simulink model "Detumbling_using_engine_sim"  (R2022b)
settings: Solver=VariableStepAuto  StartTime=0.0  StopTime=Params.tf  FixedStep=1e-2  RelTol=1e-8  AbsTol=1e-8
values from neighbouring files (symbols this model uses):
  Pitch_thrust_operator = abs(-1/( (1/(norm(Params.arm_vec1)))*(sin(gamma1)*sin(theta)*Params.arm_vec1(3)-cos(gamma1)*Params.arm_vec1(1))+         (1/(norm(Params.arm_vec2)))*(-sin(gamma2)*sin(theta)*Params.arm_vec2(3)-cos(gamma2)*Params.arm_vec2(1))+         (1/(norm(Params.arm_vec3)))*(sin(gamma3)*cos(theta)*Params.arm_vec3(3)+cos(gamma3)*Params.arm_vec3(2))+         (1/(norm(Params.arm_vec4)))*(sin(gamma4)*sin(theta)*Pa ...(+61 chars)    [Detumbling_using_engine_SimCode.m]
  Roll_thrust_operator = abs(-1/( (1/(norm(Params.arm_vec1)))*(-sin(gamma1)*cos(theta)*Params.arm_vec1(3)+cos(gamma1)*Params.arm_vec1(2))+         (1/(norm(Params.arm_vec2)))*(-sin(gamma2)*cos(theta)*Params.arm_vec2(3)+cos(gamma2)*Params.arm_vec2(2))+         (1/(norm(Params.arm_vec3)))*(sin(gamma3)*sin(theta)*Params.arm_vec3(3)-cos(gamma3)*Params.arm_vec3(1))+         (1/(norm(Params.arm_vec4)))*(sin(gamma4)*cos(theta)*P ...(+51 chars)    [Detumbling_using_engine_SimCode.m]
  tau_Thrusters = 30e-03    (= 0.03)    [Detumbling_using_engine_SimCode.m]
  w_c = [0,0,0]'    [Detumbling_using_engine_SimCode.m]
  Yaw_thrust_operator = abs(-1/( (1/(norm(Params.arm_vec1)))*(-sin(gamma1)*sin(theta)*Params.arm_vec1(2)+cos(theta)*sin(gamma1)*Params.arm_vec1(1))+         (1/(norm(Params.arm_vec2)))*(-sin(gamma2)*sin(theta)*Params.arm_vec2(2)-cos(theta)*sin(gamma2)*Params.arm_vec2(1))+         (1/(norm(Params.arm_vec3)))*(-sin(gamma3)*sin(theta)*Params.arm_vec3(2)-sin(gamma3)*cos(theta)*Params.arm_vec3(1))+         (1/(norm(Params.arm ...(+86 chars)    [Detumbling_using_engine_SimCode.m]
undefined symbols (not defined in the file or in its folder): gain, Params, Pitch, rad, Roll, s, T1, time_T1, Yaw
libraries: matrix_library x24, aerolibconvert2 x1, simulink_extras x1, sharedutil x1
(part 1 of 2)
settings Model: Creator=orena  LastModifiedBy=שקד
settings SolverCC: AlgebraicLoopSolver=TrustRegion
settings DebuggingCC: UnconnectedInputMsg=warning  UnconnectedOutputMsg=warning  UnconnectedLineMsg=warning  SFMachineParentedDataDiag=warning
settings ModelReferenceCC: EnableRefExpFcnMdlSchedulingChecks=on
settings RTWCC: DLArmComputeVersion=19.05

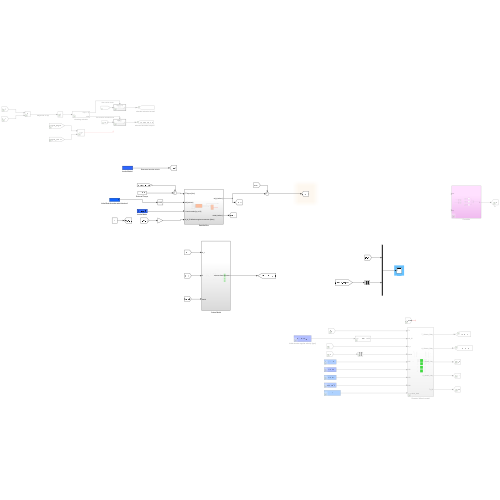
[thumbnail: Simulink's stored preview of the top-level diagram]
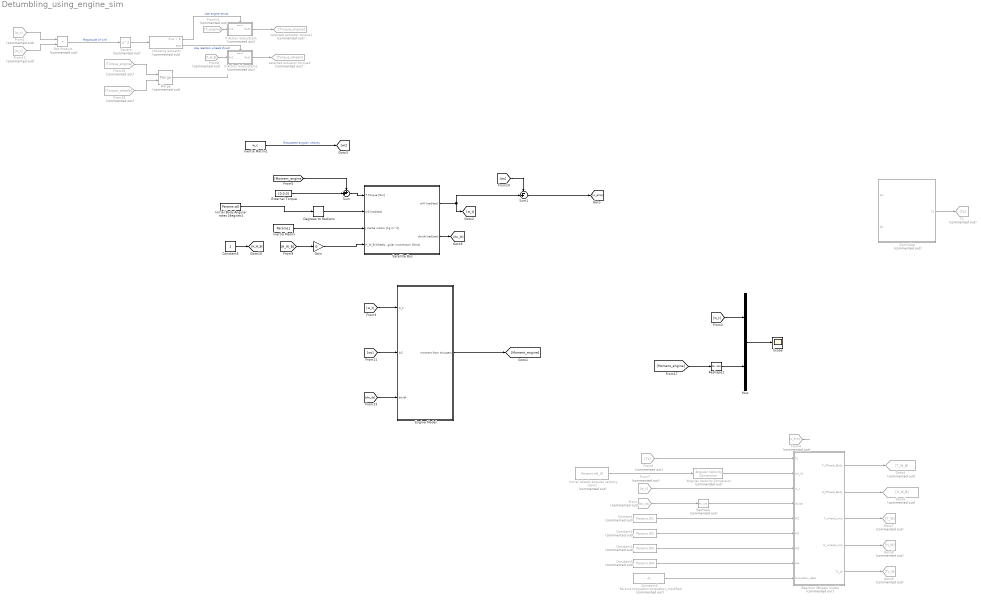
== system Detumbling_using_engine_sim ==
  Angular Velocity Conversion : aerolibconvert2/Angular Velocity Conversion  Commented=on  IU=rpm  OU=rad/s
  Constant : Constant  Commented=on  Value=Params.W1
  Constant1 : Constant  Commented=on  Value=Params.W2
  Constant2 : Constant  Commented=on  Value=Params.W3
  Constant3 : Constant  Commented=on  Value=Params.W4
  Constant4 : Constant  Commented=on  Value=Params.torquebox.torquebox_modified
  Constant5 : Constant
  Controller : Subsystem  Commented=on
  Degrees to Radians : simulink_extras/Transformations/Degrees to Radians
  Dot Product : DotProduct  Commented=on  OutDataTypeStr=Inherit: Inherit via internal rule
  Engine Model : Subsystem
  External Torque : Constant  Value=[0,0,0]
  From : From  Commented=on  GotoTag=dw_dt
  From1 : From  Commented=on  GotoTag=w_t
  From12 : From  Commented=on  GotoTag=w_t
  From14 : From  Commented=on  GotoTag=T_engine
  From15 : From  Commented=on  GotoTag=Torque_engine
  From16 : From  Commented=on  GotoTag=Torque_wheels
  From4 : From  Commented=on  GotoTag=w_error
  From6 : From  Commented=on  GotoTag=Tc
  From7 : From  Commented=on  GotoTag=w_t
  From8 : From  Commented=on  GotoTag=T_W_B
  Gain : Gain  Gain=0
  Goto4 : Goto  Commented=on  GotoTag=T_W_B
  Goto6 : Goto  Commented=on  GotoTag=H_W_B
  Goto7 : Goto  Commented=on  GotoTag=T_W
  Goto8 : Goto  Commented=on  GotoTag=H_W
  Goto9 : Goto  Commented=on  GotoTag=Tc_W
  If Action Subsystem : Subsystem  Commented=on  TreatAsAtomicUnit=on
  If Action Subsystem1 : Subsystem  Commented=on  TreatAsAtomicUnit=on
  Inertia Matrix : Constant  Value=Params.J
  Inertia Matrix1 : Constant  Value=w_c
  Initial Body Angular rates [deg/sec] : Constant  Value=Params.w0
  Initial wheels angular velocity [rpm] : Constant  Commented=on  Value=Params.w0_W
  Merge : Merge  Commented=on  InitialOutput=[0]
  Mux : Mux  Inputs=2
  Reaction Wheels model : Subsystem  Commented=on
  Reshape : Reshape  Commented=on  OutputDimensionality=Column vector (2-D)
  Reshape1 : Reshape  OutputDimensionality=Column vector (2-D)
  Satellite Bus : Subsystem
  Scope : Scope
  Square : Math  Commented=on  Operator=square
  Sum : Sum  Inputs=++|
  Sum1 : Sum  Inputs=-+|
  Tc : Goto  Commented=on  GotoTag=Tc
  choosing actuator : If  Commented=on  IfExpression=u1 > 5
  selected actuator torque1 : Goto  Commented=on  GotoTag=Torque_engine
  selected actuator torque2 : Goto  Commented=on  GotoTag=Torque_wheels
  wires:
  Initial Body Angular rates [deg/sec]/1 -> Degrees to Radians/1
  External Torque/1 -> Sum/2
  Controller/1(Tc) -> Tc/1
  From8/1 -> If Action Subsystem1/1(In1)
  [wc] -> Sum1/1
  Sum/1 -> Satellite Bus/1(T Torque [Nm])
  Degrees to Radians/1 -> Satellite Bus/2(w0 [rad/sec])
  Inertia Matrix/1 -> Satellite Bus/3(J inertia matrix [kg m^2])
  Satellite Bus/1(w(t) [rad/sec]) -> Sum1/2, [w_t]
  Sum1/1 -> [w_error]
  Mux/1 -> Scope/1
  [w_t] -> Mux/1
  From4/1 -> ?
  Angular Velocity Conversion/1 -> Reaction Wheels model/2(w0_W)
  From6/1 -> Reaction Wheels model/1(Tc)
  From7/1 -> Reaction Wheels model/3(w_t)
  Reaction Wheels model/1(T_Wheels_Body) -> Goto4/1
  Satellite Bus/2(dw/dt [rad/sec]) -> [dw_dt]
  From/1 -> Reshape/1
  Constant/1 -> Reaction Wheels model/5(W1)
  Constant1/1 -> Reaction Wheels model/6(W2)
  Constant2/1 -> Reaction Wheels model/7(W3)
  Constant3/1 -> Reaction Wheels model/8(W4)
  Reaction Wheels model/2(H_Wheels_Body) -> Goto6/1
  Reaction Wheels model/3(T_wheels_only) -> Goto7/1
  Reaction Wheels model/4(H_wheels_only) -> Goto8/1
  [H_W_B] -> Gain/1
  Constant4/1 -> Reaction Wheels model/9(torquebox_data)
  Reshape/1 -> Reaction Wheels model/4(dw/dt)
  Reaction Wheels model/5(Tc_W) -> Goto9/1
  Initial wheels angular velocity [rpm]/1 -> Angular Velocity Conversion/1
  Square/1 -> choosing actuator/1
  choosing actuator/1 -> If Action Subsystem/Action  "Use engine thrust"
  choosing actuator/2 -> If Action Subsystem1/Action  "Use reaction wheels thrust"
  From1/1 -> Dot Product/1
  From12/1 -> Dot Product/2
  Dot Product/1 -> Square/1  "Magnitude of w(t)"
  If Action Subsystem1/1(Out1) -> selected actuator torque2/1
  If Action Subsystem/1(Out1) -> selected actuator torque1/1
  Merge/1 -> ?
  From14/1 -> If Action Subsystem/1(In1)
  From15/1 -> Merge/1
  From16/1 -> Merge/2
  Gain/1 -> Satellite Bus/4(H_W_B Wheels angular momentum [Nms])
  Constant5/1 -> [H_W_B]
  [w_t] -> Engine Model/1(w_t)
  [dw_dt] -> Engine Model/3(dw/dt)
  Engine Model/1(moment from thrusters) -> [Moment_engine]
  [Moment_engine] -> Sum/1
  Inertia Matrix1/1 -> [wc]  "Requested angular velocity"
  [wc] -> Engine Model/2(In2)
  [Moment_engine] -> Reshape1/1
  Reshape1/1 -> Mux/2

== system Detumbling_using_engine_sim/Controller ==
  dw : Inport
  dq : Inport  Port=2
  Demux : Demux  Outputs=3
  Demux1 : Demux
  Mux : Mux  Inputs=3
  X_controller : Subsystem
  Y_controller : Subsystem
  Z_controller : Subsystem
  Tc : Outport
  wires:
  Demux/1 -> [dw1]
  [dw2] -> Y_controller/2(dw2)
  [dq1] -> X_controller/1(dq1)
  [dq3] -> Z_controller/1(dq3)
  Demux/2 -> [dw2]
  Demux/3 -> [dw3]
  [dw3] -> Z_controller/2(dw3)
  Demux1/3 -> [dq3]
  Demux1/1 -> [dq1]
  Demux1/2 -> [dq2]
  [dq2] -> Y_controller/1(dq2)
  dw/1 -> Demux/1
  [dw1] -> X_controller/2(dw1)
  Y_controller/1(Tcy) -> Mux/2
  X_controller/1(Tcx) -> Mux/1
  Z_controller/1(Tcz) -> Mux/3
  dq/1 -> Demux1/1
  Demux1/4 -> [dq4]
  [dq4] -> X_controller/3(dq4)
  [dq4] -> Y_controller/3(dq4)
  [dq4] -> Z_controller/3(dq4)
  Mux/1 -> Tc/1

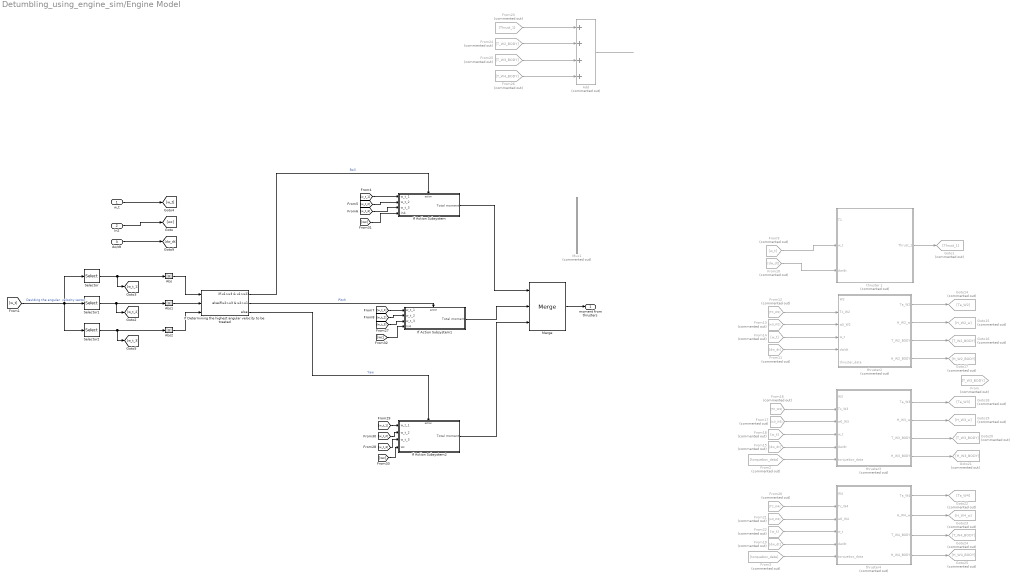
== system Detumbling_using_engine_sim/Engine Model ==
  w_t : Inport
  In2 : Inport  Port=2
  dw/dt : Inport  Port=3
  Abs : Abs  SaturateOnIntegerOverflow=off
  Abs1 : Abs  SaturateOnIntegerOverflow=off
  Abs2 : Abs  SaturateOnIntegerOverflow=off
  Add : Sum  Commented=on  Inputs=++++
  From : From  Commented=on  GotoTag=T_W3_BODY
  From{10..11,15,19} (4 alike) : From  Commented=on  GotoTag=dw_dt
  From12 : From  Commented=on  GotoTag=TC_W2
  From13 : From  Commented=on  GotoTag=w0_W2
  From{9,14,18,22} (4 alike) : From  Commented=on  GotoTag=w_t
  From16 : From  Commented=on  GotoTag=TC_W3
  From17 : From  Commented=on  GotoTag=w0_W3
  From2 : From  Commented=on  GotoTag=torquebox_data
  From20 : From  Commented=on  GotoTag=TC_W4
  From21 : From  Commented=on  GotoTag=w0_W4
  From23 : From  Commented=on  GotoTag=Thrust_1
  From24 : From  Commented=on  GotoTag=T_W2_BODY
  From25 : From  Commented=on  GotoTag=T_W3_BODY
  From26 : From  Commented=on  GotoTag=T_W4_BODY
  From3 : From  Commented=on  GotoTag=torquebox_data
  Goto1 : Goto  Commented=on  GotoTag=Thrust_1
  Goto14 : Goto  Commented=on  GotoTag=Ta_W2
  Goto15 : Goto  Commented=on  GotoTag=H_W2_w
  Goto16 : Goto  Commented=on  GotoTag=T_W2_BODY
  Goto17 : Goto  Commented=on  GotoTag=H_W2_BODY
  Goto18 : Goto  Commented=on  GotoTag=Ta_W3
  Goto19 : Goto  Commented=on  GotoTag=H_W3_w
  Goto20 : Goto  Commented=on  GotoTag=T_W3_BODY
  Goto21 : Goto  Commented=on  GotoTag=H_W3_BODY
  Goto22 : Goto  Commented=on  GotoTag=Ta_W4
  Goto23 : Goto  Commented=on  GotoTag=H_W4_w
  Goto24 : Goto  Commented=on  GotoTag=T_W4_BODY
  Goto25 : Goto  Commented=on  GotoTag=H_W4_BODY
  If Determining the highest angular velocity to be treated : If  NumInputs=3  IfExpression=u1>u3 & u1>u2  ElseIfExpressions=u2>u3 & u2>u1
  If Action Subsystem : Subsystem  TreatAsAtomicUnit=on
  If Action Subsystem1 : Subsystem  TreatAsAtomicUnit=on
  If Action Subsystem2 : Subsystem  TreatAsAtomicUnit=on
  Merge : Merge  Inputs=3
  Mux1 : Mux  Commented=on
  Selector : Selector  InputPortWidth=3  IndexOptions=Index vector (dialog)  Indices=[1]  OutputSizes=1
  Selector1 : Selector  InputPortWidth=3  IndexOptions=Index vector (dialog)  Indices=[2]  OutputSizes=1
  Selector2 : Selector  InputPortWidth=3  IndexOptions=Index vector (dialog)  Indices=[3]  OutputSizes=1
  thruster 1 : Subsystem  Commented=on
  thruster2 : Subsystem  Commented=on
  thruster3 : Subsystem  Commented=on
  thruster4 : Subsystem  Commented=on
  moment from thrusters : Outport
  wires:
  thruster2/3(T_W2_BODY) -> Goto16/1
  dw/dt/1 -> [dw_dt]
  thruster2/2(H_W2_w) -> Goto15/1
  From9/1 -> thruster 1/2(w_t)
  From22/1 -> thruster4/4(w_t)
  From12/1 -> thruster2/2(Tc_W2)
  thruster3/3(T_W3_BODY) -> Goto20/1
  From24/1 -> Add/2
  thruster2/4(H_W2_BODY) -> Goto17/1
  From15/1 -> thruster3/5(dw/dt)
  From14/1 -> thruster2/4(w_t)
  thruster4/3(T_W4_BODY) -> Goto24/1
  thruster3/2(H_W3_w) -> Goto19/1
  thruster4/4(H_W4_BODY) -> Goto25/1
  From10/1 -> thruster 1/3(dw/dt)
  thruster3/4(H_W3_BODY) -> Goto21/1
  thruster2/1(Ta_W2) -> Goto14/1
  w_t/1 -> [w_t]
  Merge/1 -> moment from thrusters/1
  thruster4/2(H_W4_w) -> Goto23/1
  From26/1 -> Add/4
  From13/1 -> thruster2/3(w0_W2)
  From19/1 -> thruster4/5(dw/dt)
  From16/1 -> thruster3/2(Tc_W3)
  From11/1 -> thruster2/5(dw/dt)
  From18/1 -> thruster3/4(w_t)
  From20/1 -> thruster4/2(Tc_W4)
  thruster 1/1(Thrust_1) -> Goto1/1
  thruster3/1(Ta_W3) -> Goto18/1
  From25/1 -> Add/3
  Add/1 -> ?
  From17/1 -> thruster3/3(w0_W3)
  From21/1 -> thruster4/3(w0_W4)
  thruster4/1(Ta_W4) -> Goto22/1
  From23/1 -> Add/1
  From2/1 -> thruster3/6(torquebox_data)
  From3/1 -> thruster4/6(torquebox_data)
  [w_t] -> Selector/1, Selector1/1, Selector2/1  "Deviding the angular  velocity vector"
  If Determining the highest angular velocity to be treated/1 -> If Action Subsystem/Action  "Roll"
  Selector/1 -> [w_t_1], Abs/1
  Abs/1 -> If Determining the highest angular velocity to be treated/1
  Abs1/1 -> If Determining the highest angular velocity to be treated/2
  Selector1/1 -> [w_t_2], Abs1/1
  Selector2/1 -> [w_t_3], Abs2/1
  Abs2/1 -> If Determining the highest angular velocity to be treated/3
  If Determining the highest angular velocity to be treated/2 -> If Action Subsystem1/Action  "Pitch"
  If Determining the highest angular velocity to be treated/3 -> If Action Subsystem2/Action  "Yaw"
  [w_t_1] -> If Action Subsystem/1(w_t_1)
  [w_t_2] -> If Action Subsystem/2(w_t_2)
  [w_t_3] -> If Action Subsystem/3(w_t_3)
  [w_t_1] -> If Action Subsystem1/1(w_t_1)
  [w_t_2] -> If Action Subsystem1/2(w_t_2)
  [w_t_3] -> If Action Subsystem1/3(w_t_3)
  [w_t_1] -> If Action Subsystem2/1(w_t_1)
  [w_t_2] -> If Action Subsystem2/2(w_t_2)
  [w_t_3] -> If Action Subsystem2/3(w_t_3)
  If Action Subsystem/1(Total moment) -> Merge/1
  If Action Subsystem1/1(Total moment) -> Merge/2
  If Action Subsystem2/1(Total moment) -> Merge/3
  In2/1 -> [wc]
  [wc] -> If Action Subsystem/4(In4)
  [wc] -> If Action Subsystem1/4(In4)
  [wc] -> If Action Subsystem2/4(wc)

== system Detumbling_using_engine_sim/If Action Subsystem ==
  In1 : Inport
  Action Port : ActionPort  ActionPortLabel=if(u1 > 5)
  Out1 : Outport
  wires:
  In1/1 -> Out1/1

== system Detumbling_using_engine_sim/If Action Subsystem1 ==
  In1 : Inport
  Action Port : ActionPort  ActionPortLabel=else
  Out1 : Outport
  wires:
  In1/1 -> Out1/1

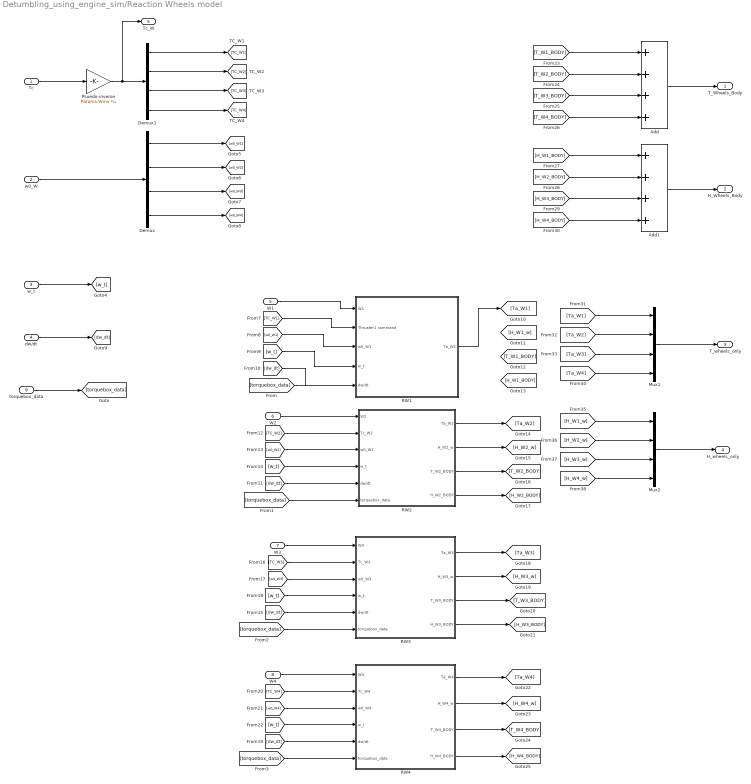
== system Detumbling_using_engine_sim/Reaction Wheels model ==
  Tc : Inport
  w0_W : Inport  Port=2
  w_t : Inport  Port=3
  dw/dt : Inport  Port=4
  W1 : Inport  Port=5
  W2 : Inport  Port=6
  W3 : Inport  Port=7
  W4 : Inport  Port=8
  torquebox_data : Inport  Port=9
  Add : Sum  Inputs=++++
  Add1 : Sum  Inputs=++++
  Demux : Demux
  Demux1 : Demux
  Mux1 : Mux
  Mux2 : Mux
  Psuedo-inverse : Gain  Gain=Params.Winv  Multiplication=Matrix(K*u) (u vector)
  RW1 : Subsystem
  RW2 : Subsystem
  RW3 : Subsystem
  RW4 : Subsystem
  T_Wheels_Body : Outport
  H_Wheels_Body : Outport  Port=2
  T_wheels_only : Outport  Port=3
  H_wheels_only : Outport  Port=4
  Tc_W : Outport  Port=5
  wires:
  RW2/3(T_W2_BODY) -> [T_W2_BODY]
  [H_W1_BODY] -> Add1/1
  W2/1 -> RW2/1(W2)
  Add1/1 -> H_Wheels_Body/1
  [TC_W1] -> RW1/2(Thruster1 command)
  Demux/3 -> [w0_W3]
  Mux2/1 -> H_wheels_only/1
  dw/dt/1 -> [dw_dt]
  Tc/1 -> Psuedo-inverse/1
  RW2/2(H_W2_w) -> [H_W2_w]
  W3/1 -> RW3/1(W3)
  w0_W/1 -> Demux/1
  [H_W2_BODY] -> Add1/2
  Psuedo-inverse/1 -> Tc_W/1, Demux1/1
  W1/1 -> RW1/1(W1)
  [w_t] -> RW1/4(w_t)
  [w_t] -> RW4/4(w_t)
  [TC_W2] -> RW2/2(Tc_W2)
  Demux1/4 -> [TC_W4]
  RW3/3(T_W3_BODY) -> [T_W3_BODY]
  ? -> [H_W1_BODY]
  [T_W2_BODY] -> Add/2
  RW2/4(H_W2_BODY) -> [H_W2_BODY]
  [Ta_W2] -> Mux1/2
  [dw_dt] -> RW3/5(dw/dt)
  [w_t] -> RW2/4(w_t)
  [H_W4_BODY] -> Add1/4
  RW4/3(T_W4_BODY) -> [T_W4_BODY]
  [H_W4_w] -> Mux2/4
  RW3/2(H_W3_w) -> [H_W3_w]
  ? -> [T_W1_BODY]
  RW4/4(H_W4_BODY) -> [H_W4_BODY]
  [dw_dt] -> RW1/5(dw/dt)
  RW3/4(H_W3_BODY) -> [H_W3_BODY]
  [Ta_W4] -> Mux1/4
  RW2/1(Ta_W2) -> [Ta_W2]
  Demux1/1 -> [TC_W1]
  [Ta_W1] -> Mux1/1
  w_t/1 -> [w_t]
  Mux1/1 -> T_wheels_only/1
  RW4/2(H_W4_w) -> [H_W4_w]
  [T_W4_BODY] -> Add/4
  Demux/4 -> [w0_W4]
  [w0_W2] -> RW2/3(w0_W2)
  [dw_dt] -> RW4/5(dw/dt)
  [TC_W3] -> RW3/2(Tc_W3)
  Demux1/3 -> [TC_W3]
  [dw_dt] -> RW2/5(dw/dt)
  W4/1 -> RW4/1(W4)
  [H_W3_w] -> Mux2/3
  ? -> [H_W1_w]
  [w_t] -> RW3/4(w_t)
  [TC_W4] -> RW4/2(Tc_W4)
  [w0_W1] -> RW1/3(w0_W1)
  RW1/1(Ta_W1) -> [Ta_W1]
  Demux/1 -> [w0_W1]
  RW3/1(Ta_W3) -> [Ta_W3]
  Demux1/2 -> [TC_W2]
  Demux/2 -> [w0_W2]
  [T_W3_BODY] -> Add/3
  [H_W1_w] -> Mux2/1
  Add/1 -> T_Wheels_Body/1
  [w0_W3] -> RW3/3(w0_W3)
  [w0_W4] -> RW4/3(w0_W4)
  RW4/1(Ta_W4) -> [Ta_W4]
  [H_W2_w] -> Mux2/2
  [H_W3_BODY] -> Add1/3
  [T_W1_BODY] -> Add/1
  [Ta_W3] -> Mux1/3
  torquebox_data/1 -> [torquebox_data]
  [torquebox_data] -> ?
  [torquebox_data] -> RW2/6(torquebox_data)
  [torquebox_data] -> RW3/6(torquebox_data)
  [torquebox_data] -> RW4/6(torquebox_data)

== system Detumbling_using_engine_sim/Satellite Bus ==
  T Torque [Nm] : Inport
  w0 [rad/sec] : Inport  Port=2
  J inertia matrix [kg m^2] : Inport  Port=3
  H_W_B Wheels angular momentum [Nms] : Inport  Port=4
  Satellite Dynamics : Subsystem
  Satellite Kinematics : Subsystem  Commented=on
  w(t) [rad/sec] : Outport
  dw/dt [rad/sec] : Outport  Port=2
  wires:
  Satellite Kinematics/1(q(t)) -> ?
  J inertia matrix [kg m^2]/1 -> Satellite Dynamics/3(J inertia matrix [kg m^2])
  w0 [rad/sec]/1 -> Satellite Dynamics/2(w0 [rad/sec])
  Satellite Dynamics/1(w(t) [rad/sec]) -> Satellite Kinematics/1(w(t) [rad/sec]), w(t) [rad/sec]/1
  T Torque [Nm]/1 -> Satellite Dynamics/1(T Torque [Nm])
  Satellite Dynamics/2(dw/dt [rad/sec^2]) -> dw/dt [rad/sec]/1
  H_W_B Wheels angular momentum [Nms]/1 -> Satellite Dynamics/4(H_W_B Wheels angular momentum [Nms])

== system Detumbling_using_engine_sim/Controller/X_controller ==
  dq1 : Inport
  dw1 : Inport  Port=2
  dq4 : Inport  Port=3
  Gain : Gain  Gain=Params.gains.kdx
  Gain1 : Gain  Gain=Params.gains.kpx
  Product : Product
  Sign : Signum
  Sum2 : Sum  Inputs=+|+
  Tcx : Outport
  wires:
  Sum2/1 -> Tcx/1
  dq1/1 -> Gain1/1
  dw1/1 -> Gain/1
  Gain/1 -> Sum2/2
  dq4/1 -> Sign/1
  Sign/1 -> Product/1
  Gain1/1 -> Product/2
  Product/1 -> Sum2/1

== system Detumbling_using_engine_sim/Controller/Y_controller ==
  dq2 : Inport
  dw2 : Inport  Port=2
  dq4 : Inport  Port=3
  Gain2 : Gain  Gain=Params.gains.kpy
  Gain3 : Gain  Gain=Params.gains.kdy
  Product : Product
  Sign : Signum
  Sum3 : Sum  Inputs=+|+
  Tcy : Outport
  wires:
  dq2/1 -> Gain2/1
  Gain3/1 -> Sum3/2
  Sum3/1 -> Tcy/1
  dw2/1 -> Gain3/1
  dq4/1 -> Sign/1
  Sign/1 -> Product/1
  Gain2/1 -> Product/2
  Product/1 -> Sum3/1

== system Detumbling_using_engine_sim/Controller/Z_controller ==
  dq3 : Inport
  dw3 : Inport  Port=2
  dq4 : Inport  Port=3
  Gain4 : Gain  Gain=Params.gains.kpz
  Gain5 : Gain  Gain=Params.gains.kdz
  Product : Product
  Sign : Signum
  Sum4 : Sum  Inputs=+|+
  Tcz : Outport
  wires:
  Sum4/1 -> Tcz/1
  dw3/1 -> Gain5/1
  Gain5/1 -> Sum4/2
  dq3/1 -> Gain4/1
  dq4/1 -> Sign/1
  Sign/1 -> Product/1
  Gain4/1 -> Product/2
  Product/1 -> Sum4/1

== system Detumbling_using_engine_sim/Engine Model/If Action Subsystem ==
  w_t_1 : Inport
  w_t_2 : Inport  Port=2
  w_t_3 : Inport  Port=3
  In4 : Inport  Port=4
  Action Port : ActionPort  ActionPortLabel=if(u1>u3 & u1>u2)
  From1 : From  Commented=on  GotoTag=w_t_2
  From2 : From  Commented=on  GotoTag=w_t_3
  From4 : From  Commented=on  GotoTag=w_t_2
  From5 : From  Commented=on  GotoTag=w_t_3
  If : If
  If Action Subsystem Roll + : Subsystem  TreatAsAtomicUnit=on
  If Action Subsystem Roll - : Subsystem  TreatAsAtomicUnit=on
  Merge : Merge
  Total moment : Outport
  wires:
  w_t_1/1 -> [w_t_1], If/1
  If/2 -> If Action Subsystem Roll -/Action  "Roll -"
  If/1 -> If Action Subsystem Roll +/Action  "Roll +"
  w_t_2/1 -> [w_t_2]
  w_t_3/1 -> [w_t_3]
  [w_t_1] -> If Action Subsystem Roll +/1(w_t_1)
  If Action Subsystem Roll +/1(Out1) -> Merge/1
  [w_t_1] -> If Action Subsystem Roll -/1(w_t_1)
  If Action Subsystem Roll -/1(Out1) -> Merge/2
  Merge/1 -> Total moment/1
  In4/1 -> [wc]
  [wc] -> If Action Subsystem Roll +/2(wc)
  [wc] -> If Action Subsystem Roll -/2(wc)

== system Detumbling_using_engine_sim/Engine Model/If Action Subsystem1 ==
  w_t_1 : Inport
  w_t_2 : Inport  Port=2
  w_t_3 : Inport  Port=3
  In4 : Inport  Port=4
  Action Port : ActionPort  ActionPortLabel=elseif(u2>u3 & u2>u1 )
  From1 : From  Commented=on  GotoTag=w_t_2
  From2 : From  Commented=on  GotoTag=w_t_3
  From4 : From  Commented=on  GotoTag=w_t_2
  From5 : From  Commented=on  GotoTag=w_t_3
  If : If
  If Action Subsystem Pitch + : Subsystem  TreatAsAtomicUnit=on
  If Action Subsystem Pitch - : Subsystem  TreatAsAtomicUnit=on
  Merge : Merge
  Total moment : Outport
  wires:
  w_t_1/1 -> [w_t_1]
  If/2 -> If Action Subsystem Pitch -/Action  "Yaw -"
  If/1 -> If Action Subsystem Pitch +/Action  "Yaw +"
  w_t_2/1 -> If/1, [w_t_2]
  w_t_3/1 -> [w_t_3]
  [w_t_1] -> If Action Subsystem Pitch +/1(w_t_1)
  If Action Subsystem Pitch +/1("Total moment generated ") -> Merge/1
  [w_t_1] -> If Action Subsystem Pitch -/1(w_t_1)
  If Action Subsystem Pitch -/1("Total moment generated ") -> Merge/2
  Merge/1 -> Total moment/1
  In4/1 -> [wc]
  [wc] -> If Action Subsystem Pitch +/4(In4)
  [wc] -> If Action Subsystem Pitch -/4(wc)

== system Detumbling_using_engine_sim/Engine Model/If Action Subsystem2 ==
  w_t_1 : Inport
  w_t_2 : Inport  Port=2
  w_t_3 : Inport  Port=3
  wc : Inport  Port=4
  Action Port : ActionPort  ActionPortLabel=else
  If : If
  If Action Subsystem Yaw + : Subsystem  TreatAsAtomicUnit=on
  If Action Subsystem Yaw - : Subsystem  TreatAsAtomicUnit=on
  Merge : Merge
  Total moment : Outport
  wires:
  w_t_2/1 -> [w_t_2]
  w_t_1/1 -> [w_t_1]
  If/1 -> If Action Subsystem Yaw +/Action  "Yaw +"
  [w_t_1] -> If Action Subsystem Yaw -/1(w_t_1)
  If Action Subsystem Yaw -/1("Total moment generated ") -> Merge/2
  [w_t_1] -> If Action Subsystem Yaw +/1(w_t_1)
  [w_t_2] -> If Action Subsystem Yaw -/2(w_t_2)
  If Action Subsystem Yaw +/1("Total moment generated ") -> Merge/1
  [w_t_3] -> If Action Subsystem Yaw +/3(w_t_3)
  If/2 -> If Action Subsystem Yaw -/Action  "Yaw -"
  [w_t_2] -> If Action Subsystem Yaw +/2(w_t_2)
  [w_t_3] -> If Action Subsystem Yaw -/3(w_t_3)
  w_t_3/1 -> [w_t_3], If/1
  Merge/1 -> Total moment/1
  wc/1 -> [wc]
  [wc] -> If Action Subsystem Yaw +/4(wc)
  [wc] -> If Action Subsystem Yaw -/4(wc)

== system Detumbling_using_engine_sim/Engine Model/thruster 1 ==
  T1 : Inport
  w_t : Inport  Port=2
  dw/dt : Inport  Port=3
  Step1 : Step  Time=7.5/T1  SampleTime=0
  Sum : Sum  Inputs=|+-
  "Time constant - open thruster " : TransferFcn  Denominator=[tau_Thrusters 1]
  Thrust_1 : Outport
  wires:
  Step1/1 -> Sum/2
  "Time constant - open thruster "/1 -> Sum/1
  Sum/1 -> [Thrust_1]
  T1/1 -> "Time constant - open thruster "/1

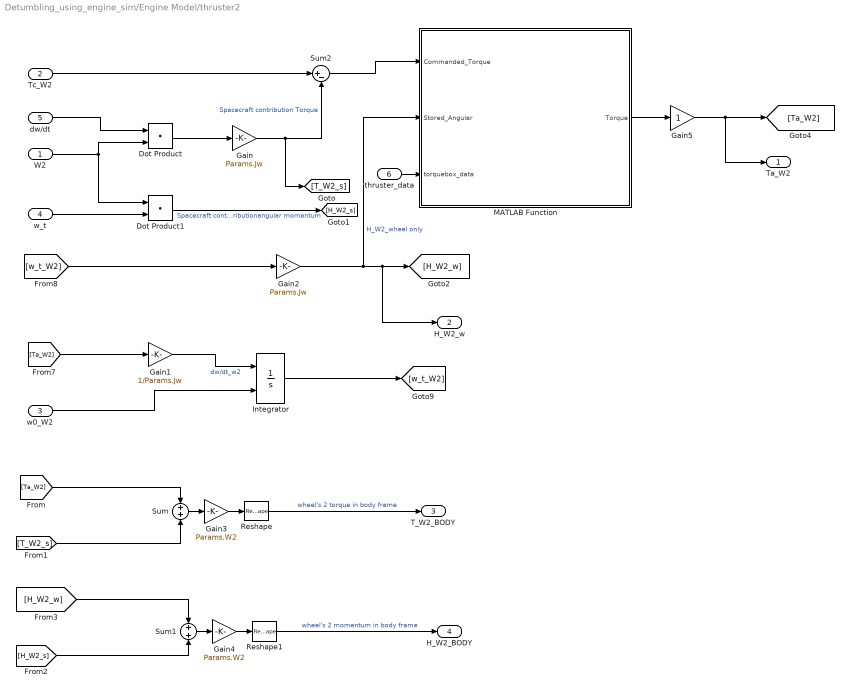
== system Detumbling_using_engine_sim/Engine Model/thruster2 ==
  W2 : Inport
  Tc_W2 : Inport  Port=2
  w0_W2 : Inport  Port=3
  w_t : Inport  Port=4
  dw/dt : Inport  Port=5
  thruster_data : Inport  Port=6
  Dot Product : DotProduct  OutDataTypeStr=Inherit: Inherit via internal rule
  Dot Product1 : DotProduct  OutDataTypeStr=Inherit: Inherit via internal rule
  Gain : Gain  Gain=Params.Jw
  Gain1 : Gain  Gain=1/Params.Jw
  Gain2 : Gain  Gain=Params.Jw
  Gain3 : Gain  Gain=Params.W2
  Gain4 : Gain  Gain=Params.W2
  Gain5 : Gain
  Integrator : Integrator  InitialConditionSource=external
  MATLAB Function : MATLAB Function  TreatAsAtomicUnit=on
  Reshape : Reshape  OutputDimensionality=Column vector (2-D)
  Reshape1 : Reshape  OutputDimensionality=Column vector (2-D)
  Sum : Sum  Inputs=+|+
  Sum1 : Sum  Inputs=+|+
  Sum2 : Sum  Inputs=|+-
  Ta_W2 : Outport
  H_W2_w : Outport  Port=2
  T_W2_BODY : Outport  Port=3
  H_W2_BODY : Outport  Port=4
  wires:
  Gain4/1 -> Reshape1/1
  Gain3/1 -> Reshape/1
  Sum1/1 -> Gain4/1
  [H_W2_w] -> Sum1/1
  [H_W2_s] -> Sum1/2
  Sum/1 -> Gain3/1
  [T_W2_s] -> Sum/2
  [Ta_W2] -> Sum/1
  Dot Product1/1 -> [H_W2_s]  "Spacecraft contributionangular momentum"
  w_t/1 -> Dot Product1/2
  [w_t_W2] -> Gain2/1
  Gain1/1 -> Integrator/1  "dw/dt_w2"
  Integrator/1 -> [w_t_W2]
  [Ta_W2] -> Gain1/1
  Gain2/1 -> MATLAB Function/2(Stored_Angular), [H_W2_w], H_W2_w/1  "H_W2_wheel only"
  Dot Product/1 -> Gain/1
  W2/1 -> Dot Product/2, Dot Product1/1
  Sum2/1 -> MATLAB Function/1(Commanded_Torque)
  w0_W2/1 -> Integrator/2
  dw/dt/1 -> Dot Product/1
  Gain/1 -> [T_W2_s], Sum2/2  "Spacecraft contribution Torque"
  Tc_W2/1 -> Sum2/1
  Reshape/1 -> T_W2_BODY/1  "wheel's 2 torque in body frame"
  Reshape1/1 -> H_W2_BODY/1  "wheel's 2 momentum in body frame"
  thruster_data/1 -> MATLAB Function/3(torquebox_data)
  MATLAB Function/1(Torque) -> Gain5/1
  Gain5/1 -> Ta_W2/1, [Ta_W2]

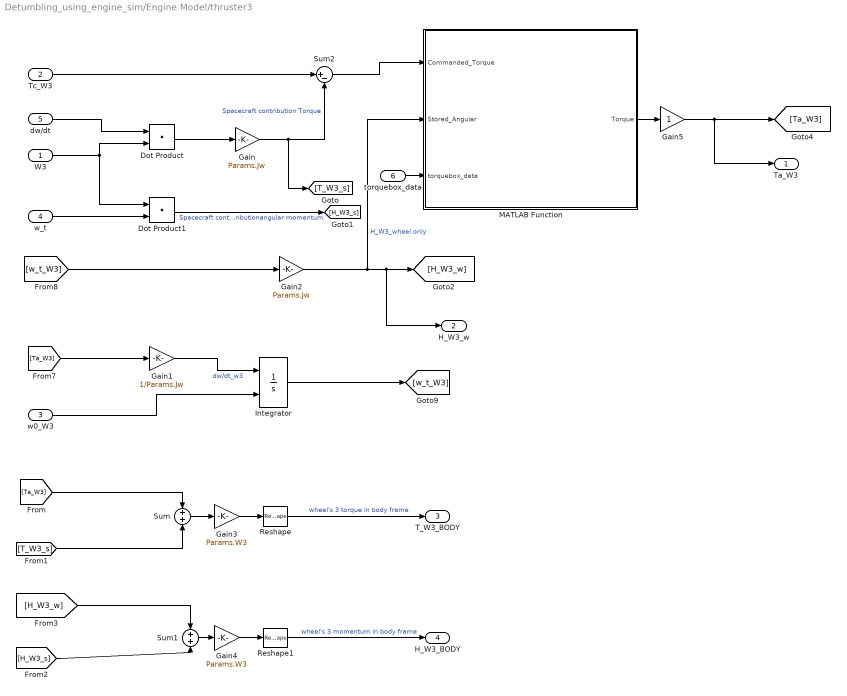
== system Detumbling_using_engine_sim/Engine Model/thruster3 ==
  W3 : Inport
  Tc_W3 : Inport  Port=2
  w0_W3 : Inport  Port=3
  w_t : Inport  Port=4
  dw/dt : Inport  Port=5
  torquebox_data : Inport  Port=6
  Dot Product : DotProduct  OutDataTypeStr=Inherit: Inherit via internal rule
  Dot Product1 : DotProduct  OutDataTypeStr=Inherit: Inherit via internal rule
  Gain : Gain  Gain=Params.Jw
  Gain1 : Gain  Gain=1/Params.Jw
  Gain2 : Gain  Gain=Params.Jw
  Gain3 : Gain  Gain=Params.W3
  Gain4 : Gain  Gain=Params.W3
  Gain5 : Gain
  Integrator : Integrator  InitialConditionSource=external
  MATLAB Function : MATLAB Function  TreatAsAtomicUnit=on
  Reshape : Reshape  OutputDimensionality=Column vector (2-D)
  Reshape1 : Reshape  OutputDimensionality=Column vector (2-D)
  Sum : Sum  Inputs=+|+
  Sum1 : Sum  Inputs=+|+
  Sum2 : Sum  Inputs=|+-
  Ta_W3 : Outport
  H_W3_w : Outport  Port=2
  T_W3_BODY : Outport  Port=3
  H_W3_BODY : Outport  Port=4
  wires:
  Tc_W3/1 -> Sum2/1
  Gain/1 -> Sum2/2, [T_W3_s]  "Spacecraft contribution Torque"
  dw/dt/1 -> Dot Product/1
  w0_W3/1 -> Integrator/2
  Sum2/1 -> MATLAB Function/1(Commanded_Torque)
  W3/1 -> Dot Product1/1, Dot Product/2
  Dot Product/1 -> Gain/1
  Gain2/1 -> H_W3_w/1, [H_W3_w], MATLAB Function/2(Stored_Angular)  "H_W3_wheel only"
  [Ta_W3] -> Gain1/1
  Integrator/1 -> [w_t_W3]
  Gain1/1 -> Integrator/1  "dw/dt_w3"
  [w_t_W3] -> Gain2/1
  w_t/1 -> Dot Product1/2
  Dot Product1/1 -> [H_W3_s]  "Spacecraft contributionangular momentum"
  [Ta_W3] -> Sum/1
  [T_W3_s] -> Sum/2
  Sum/1 -> Gain3/1
  [H_W3_s] -> Sum1/2
  [H_W3_w] -> Sum1/1
  Sum1/1 -> Gain4/1
  Gain3/1 -> Reshape/1
  Gain4/1 -> Reshape1/1
  Reshape/1 -> T_W3_BODY/1  "wheel's 3 torque in body frame"
  Reshape1/1 -> H_W3_BODY/1  "wheel's 3 momentum in body frame"
  torquebox_data/1 -> MATLAB Function/3(torquebox_data)
  MATLAB Function/1(Torque) -> Gain5/1
  Gain5/1 -> Ta_W3/1, [Ta_W3]

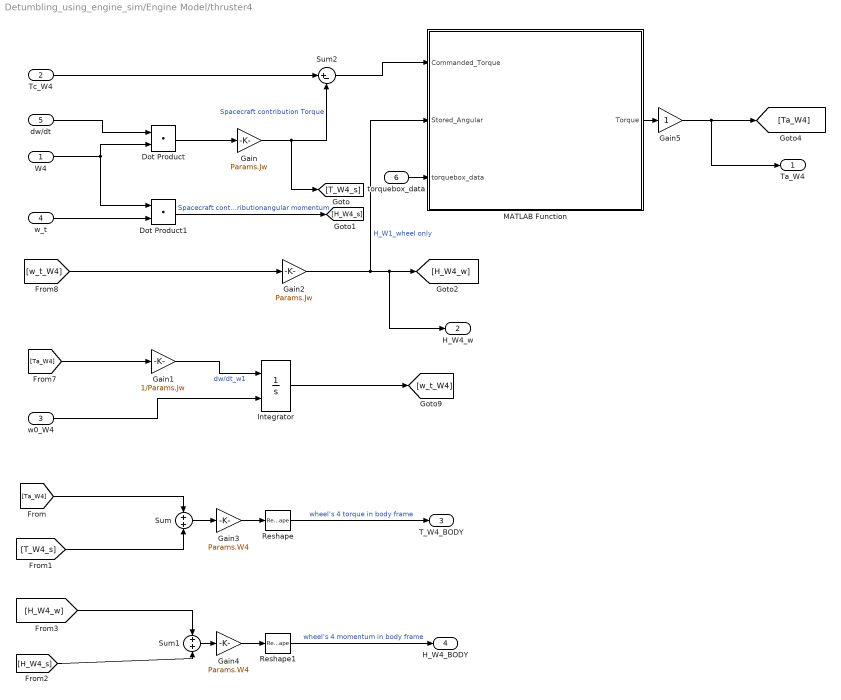
== system Detumbling_using_engine_sim/Engine Model/thruster4 ==
  W4 : Inport
  Tc_W4 : Inport  Port=2
  w0_W4 : Inport  Port=3
  w_t : Inport  Port=4
  dw/dt : Inport  Port=5
  torquebox_data : Inport  Port=6
  Dot Product : DotProduct  OutDataTypeStr=Inherit: Inherit via internal rule
  Dot Product1 : DotProduct  OutDataTypeStr=Inherit: Inherit via internal rule
  Gain : Gain  Gain=Params.Jw
  Gain1 : Gain  Gain=1/Params.Jw
  Gain2 : Gain  Gain=Params.Jw
  Gain3 : Gain  Gain=Params.W4
  Gain4 : Gain  Gain=Params.W4
  Gain5 : Gain
  Integrator : Integrator  InitialConditionSource=external
  MATLAB Function : MATLAB Function  TreatAsAtomicUnit=on
  Reshape : Reshape  OutputDimensionality=Column vector (2-D)
  Reshape1 : Reshape  OutputDimensionality=Column vector (2-D)
  Sum : Sum  Inputs=+|+
  Sum1 : Sum  Inputs=+|+
  Sum2 : Sum  Inputs=|+-
  Ta_W4 : Outport
  H_W4_w : Outport  Port=2
  T_W4_BODY : Outport  Port=3
  H_W4_BODY : Outport  Port=4
  wires:
  Gain4/1 -> Reshape1/1
  Gain3/1 -> Reshape/1
  Sum1/1 -> Gain4/1
  [H_W4_w] -> Sum1/1
  [H_W4_s] -> Sum1/2
  Sum/1 -> Gain3/1
  [T_W4_s] -> Sum/2
  [Ta_W4] -> Sum/1
  Dot Product1/1 -> [H_W4_s]  "Spacecraft contributionangular momentum"
  w_t/1 -> Dot Product1/2
  [w_t_W4] -> Gain2/1
  Gain1/1 -> Integrator/1  "dw/dt_w1"
  Integrator/1 -> [w_t_W4]
  [Ta_W4] -> Gain1/1
  Gain2/1 -> MATLAB Function/2(Stored_Angular), [H_W4_w], H_W4_w/1  "H_W1_wheel only"
  Dot Product/1 -> Gain/1
  W4/1 -> Dot Product/2, Dot Product1/1
  Sum2/1 -> MATLAB Function/1(Commanded_Torque)
  w0_W4/1 -> Integrator/2
  dw/dt/1 -> Dot Product/1
  Gain/1 -> [T_W4_s], Sum2/2  "Spacecraft contribution Torque"
  Tc_W4/1 -> Sum2/1
  Reshape/1 -> T_W4_BODY/1  "wheel's 4 torque in body frame"
  Reshape1/1 -> H_W4_BODY/1  "wheel's 4 momentum in body frame"
  torquebox_data/1 -> MATLAB Function/3(torquebox_data)
  MATLAB Function/1(Torque) -> Gain5/1
  Gain5/1 -> Ta_W4/1, [Ta_W4]

== system Detumbling_using_engine_sim/Reaction Wheels model/RW1 ==
  W1 : Inport
  Thruster1 command : Inport  Port=2
  w0_W1 : Inport  Port=3
  w_t : Inport  Port=4
  dw/dt : Inport  Port=5
  Step1 : Step  Time=time_T1  SampleTime=0
  Sum : Sum  Inputs=|+-
  "Time constant - open thruster " : TransferFcn  Denominator=[tau_Thrusters 1]
  Ta_W1 : Outport
  wires:
  Thruster1 command/1 -> "Time constant - open thruster "/1  "Force command"
  Step1/1 -> Sum/2
  "Time constant - open thruster "/1 -> Sum/1
  Sum/1 -> [Ta_W1]

== system Detumbling_using_engine_sim/Reaction Wheels model/RW2 ==
  W2 : Inport
  Tc_W2 : Inport  Port=2
  w0_W2 : Inport  Port=3
  w_t : Inport  Port=4
  dw/dt : Inport  Port=5
  torquebox_data : Inport  Port=6
  Dot Product : DotProduct  OutDataTypeStr=Inherit: Inherit via internal rule
  Dot Product1 : DotProduct  OutDataTypeStr=Inherit: Inherit via internal rule
  Gain : Gain  Gain=Params.Jw
  Gain1 : Gain  Gain=1/Params.Jw
  Gain2 : Gain  Gain=Params.Jw
  Gain3 : Gain  Gain=Params.W2
  Gain4 : Gain  Gain=Params.W2
  Gain5 : Gain
  Integrator : Integrator  InitialConditionSource=external
  MATLAB Function : MATLAB Function  TreatAsAtomicUnit=on
  Reshape : Reshape  OutputDimensionality=Column vector (2-D)
  Reshape1 : Reshape  OutputDimensionality=Column vector (2-D)
  Sum : Sum  Inputs=+|+
  Sum1 : Sum  Inputs=+|+
  Sum2 : Sum  Inputs=|+-
  Ta_W2 : Outport
  H_W2_w : Outport  Port=2
  T_W2_BODY : Outport  Port=3
  H_W2_BODY : Outport  Port=4
  wires:
  Gain4/1 -> Reshape1/1
  Gain3/1 -> Reshape/1
  Sum1/1 -> Gain4/1
  [H_W2_w] -> Sum1/1
  [H_W2_s] -> Sum1/2
  Sum/1 -> Gain3/1
  [T_W2_s] -> Sum/2
  [Ta_W2] -> Sum/1
  Dot Product1/1 -> [H_W2_s]  "Spacecraft contributionangular momentum"
  w_t/1 -> Dot Product1/2
  [w_t_W2] -> Gain2/1
  Gain1/1 -> Integrator/1  "dw/dt_w2"
  Integrator/1 -> [w_t_W2]
  [Ta_W2] -> Gain1/1
  Gain2/1 -> MATLAB Function/2(Stored_Angular), [H_W2_w], H_W2_w/1  "H_W2_wheel only"
  Dot Product/1 -> Gain/1
  W2/1 -> Dot Product/2, Dot Product1/1
  Sum2/1 -> MATLAB Function/1(Commanded_Torque)
  w0_W2/1 -> Integrator/2
  dw/dt/1 -> Dot Product/1
  Gain/1 -> [T_W2_s], Sum2/2  "Spacecraft contribution Torque"
  Tc_W2/1 -> Sum2/1
  Reshape/1 -> T_W2_BODY/1  "wheel's 2 torque in body frame"
  Reshape1/1 -> H_W2_BODY/1  "wheel's 2 momentum in body frame"
  torquebox_data/1 -> MATLAB Function/3(torquebox_data)
  MATLAB Function/1(Torque) -> Gain5/1
  Gain5/1 -> Ta_W2/1, [Ta_W2]

== system Detumbling_using_engine_sim/Reaction Wheels model/RW3 ==
  W3 : Inport
  Tc_W3 : Inport  Port=2
  w0_W3 : Inport  Port=3
  w_t : Inport  Port=4
  dw/dt : Inport  Port=5
  torquebox_data : Inport  Port=6
  Dot Product : DotProduct  OutDataTypeStr=Inherit: Inherit via internal rule
  Dot Product1 : DotProduct  OutDataTypeStr=Inherit: Inherit via internal rule
  Gain : Gain  Gain=Params.Jw
  Gain1 : Gain  Gain=1/Params.Jw
  Gain2 : Gain  Gain=Params.Jw
  Gain3 : Gain  Gain=Params.W3
  Gain4 : Gain  Gain=Params.W3
  Gain5 : Gain
  Integrator : Integrator  InitialConditionSource=external
  MATLAB Function : MATLAB Function  TreatAsAtomicUnit=on
  Reshape : Reshape  OutputDimensionality=Column vector (2-D)
  Reshape1 : Reshape  OutputDimensionality=Column vector (2-D)
  Sum : Sum  Inputs=+|+
  Sum1 : Sum  Inputs=+|+
  Sum2 : Sum  Inputs=|+-
  Ta_W3 : Outport
  H_W3_w : Outport  Port=2
  T_W3_BODY : Outport  Port=3
  H_W3_BODY : Outport  Port=4
  wires:
  Tc_W3/1 -> Sum2/1
  Gain/1 -> Sum2/2, [T_W3_s]  "Spacecraft contribution Torque"
  dw/dt/1 -> Dot Product/1
  w0_W3/1 -> Integrator/2
  Sum2/1 -> MATLAB Function/1(Commanded_Torque)
  W3/1 -> Dot Product1/1, Dot Product/2
  Dot Product/1 -> Gain/1
  Gain2/1 -> H_W3_w/1, [H_W3_w], MATLAB Function/2(Stored_Angular)  "H_W3_wheel only"
  [Ta_W3] -> Gain1/1
  Integrator/1 -> [w_t_W3]
  Gain1/1 -> Integrator/1  "dw/dt_w3"
  [w_t_W3] -> Gain2/1
  w_t/1 -> Dot Product1/2
  Dot Product1/1 -> [H_W3_s]  "Spacecraft contributionangular momentum"
  [Ta_W3] -> Sum/1
  [T_W3_s] -> Sum/2
  Sum/1 -> Gain3/1
  [H_W3_s] -> Sum1/2
  [H_W3_w] -> Sum1/1
  Sum1/1 -> Gain4/1
  Gain3/1 -> Reshape/1
  Gain4/1 -> Reshape1/1
  Reshape/1 -> T_W3_BODY/1  "wheel's 3 torque in body frame"
  Reshape1/1 -> H_W3_BODY/1  "wheel's 3 momentum in body frame"
  torquebox_data/1 -> MATLAB Function/3(torquebox_data)
  MATLAB Function/1(Torque) -> Gain5/1
  Gain5/1 -> Ta_W3/1, [Ta_W3]

== system Detumbling_using_engine_sim/Reaction Wheels model/RW4 ==
  W4 : Inport
  Tc_W4 : Inport  Port=2
  w0_W4 : Inport  Port=3
  w_t : Inport  Port=4
  dw/dt : Inport  Port=5
  torquebox_data : Inport  Port=6
  Dot Product : DotProduct  OutDataTypeStr=Inherit: Inherit via internal rule
  Dot Product1 : DotProduct  OutDataTypeStr=Inherit: Inherit via internal rule
  Gain : Gain  Gain=Params.Jw
  Gain1 : Gain  Gain=1/Params.Jw
  Gain2 : Gain  Gain=Params.Jw
  Gain3 : Gain  Gain=Params.W4
  Gain4 : Gain  Gain=Params.W4
  Gain5 : Gain
  Integrator : Integrator  InitialConditionSource=external
  MATLAB Function : MATLAB Function  TreatAsAtomicUnit=on
  Reshape : Reshape  OutputDimensionality=Column vector (2-D)
  Reshape1 : Reshape  OutputDimensionality=Column vector (2-D)
  Sum : Sum  Inputs=+|+
  Sum1 : Sum  Inputs=+|+
  Sum2 : Sum  Inputs=|+-
  Ta_W4 : Outport
  H_W4_w : Outport  Port=2
  T_W4_BODY : Outport  Port=3
  H_W4_BODY : Outport  Port=4
  wires:
  Gain4/1 -> Reshape1/1
  Gain3/1 -> Reshape/1
  Sum1/1 -> Gain4/1
  [H_W4_w] -> Sum1/1
  [H_W4_s] -> Sum1/2
  Sum/1 -> Gain3/1
  [T_W4_s] -> Sum/2
  [Ta_W4] -> Sum/1
  Dot Product1/1 -> [H_W4_s]  "Spacecraft contributionangular momentum"
  w_t/1 -> Dot Product1/2
  [w_t_W4] -> Gain2/1
  Gain1/1 -> Integrator/1  "dw/dt_w1"
  Integrator/1 -> [w_t_W4]
  [Ta_W4] -> Gain1/1
  Gain2/1 -> MATLAB Function/2(Stored_Angular), [H_W4_w], H_W4_w/1  "H_W1_wheel only"
  Dot Product/1 -> Gain/1
  W4/1 -> Dot Product/2, Dot Product1/1
  Sum2/1 -> MATLAB Function/1(Commanded_Torque)
  w0_W4/1 -> Integrator/2
  dw/dt/1 -> Dot Product/1
  Gain/1 -> [T_W4_s], Sum2/2  "Spacecraft contribution Torque"
  Tc_W4/1 -> Sum2/1
  Reshape/1 -> T_W4_BODY/1  "wheel's 4 torque in body frame"
  Reshape1/1 -> H_W4_BODY/1  "wheel's 4 momentum in body frame"
  torquebox_data/1 -> MATLAB Function/3(torquebox_data)
  MATLAB Function/1(Torque) -> Gain5/1
  Gain5/1 -> Ta_W4/1, [Ta_W4]

== system Detumbling_using_engine_sim/Satellite Bus/Satellite Dynamics ==
  T Torque [Nm] : Inport
  w0 [rad/sec] : Inport  Port=2
  J inertia matrix [kg m^2] : Inport  Port=3
  H_W_B Wheels angular momentum [Nms] : Inport  Port=4
  Add : Sum
  Add1 : Sum
  From3 : From
  Gain : Gain  Gain=-1
  Goto1 : Goto
  H=Jw : Product  Multiplication=Matrix(*)
  Integrator : Integrator  InitialConditionSource=external
  Matrix Divide : Product  Inputs=*/  Multiplication=Matrix(*)
  Reshape : Reshape  OutputDimensionality=Row vector (2-D)
  Transpose : Math  Operator=transpose
  wXH : sharedutil/3x3 Cross Product  aMode=aMode
  w(t) [rad/sec] : Outport
  dw/dt [rad/sec^2] : Outport  Port=2
  wires:
  T Torque [Nm]/1 -> Add/2
  w0 [rad/sec]/1 -> Integrator/2
  Gain/1 -> Add/1
  [w_t] -> w(t) [rad/sec]/1
  J inertia matrix [kg m^2]/1 -> Matrix Divide/2, H=Jw/1
  [dwdt] -> Integrator/1
  wXH/1 -> Gain/1
  [w_t] -> wXH/1
  From3/1 -> Reshape/1
  Matrix Divide/1 -> [dwdt]
  [w_t] -> H=Jw/2
  Integrator/1 -> Transpose/1
  Transpose/1 -> [w_t]
  [dwdt] -> dw/dt [rad/sec^2]/1
  H_W_B Wheels angular momentum [Nms]/1 -> Add1/2
  Add/1 -> Goto1/1
  H=Jw/1 -> Add1/1
  Add1/1 -> wXH/2
  Reshape/1 -> Matrix Divide/1

== system Detumbling_using_engine_sim/Satellite Bus/Satellite Kinematics ==
  w(t) [rad/sec] : Inport
  CHI(q) : Subsystem
  Gain : Gain  Gain=1/2
  Integrator : Integrator  InitialConditionSource=external
  MATLAB Function1 : MATLAB Function  Commented=on  TreatAsAtomicUnit=on
  Matrix Multiply : Product  Multiplication=Matrix(*)
  q(t) : Outport
  wires:
  [dqdt] -> Integrator/1
  [q_t] -> q(t)/1
  Gain/1 -> [dqdt]
  Integrator/1 -> [q_t]
  Matrix Multiply/1 -> Gain/1
  w(t) [rad/sec]/1 -> Matrix Multiply/2
  CHI(q)/1(CHI) -> Matrix Multiply/1
  [q_t] -> CHI(q)/1(q)

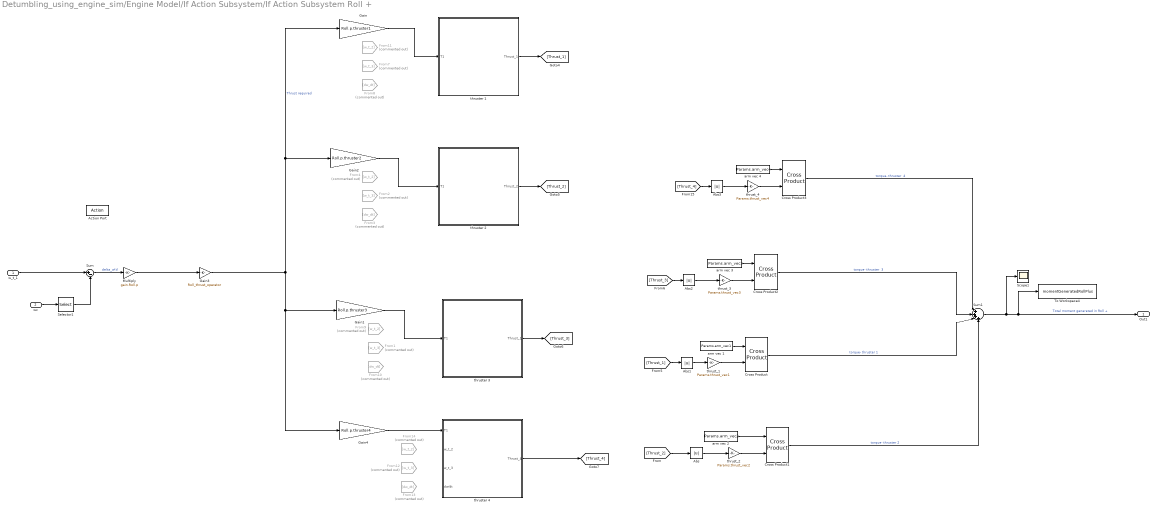
== system Detumbling_using_engine_sim/Engine Model/If Action Subsystem/If Action Subsystem Roll + ==
  w_t_1 : Inport
  wc : Inport  Port=2
  Action Port : ActionPort  ActionPortLabel=if(u1 > 0)
  Abs{,1..3} (4 alike) : Abs  SaturateOnIntegerOverflow=off
  Cross Product{,1..3} (4 alike) : matrix_library/Cross Product
  From{1..2,7,12} (4 alike) : From  Commented=on  GotoTag=w_t_3
  From{3,8,10,13} (4 alike) : From  Commented=on  GotoTag=dw_dt
  From{4,9,11,14} (4 alike) : From  Commented=on  GotoTag=w_t_2
  Gain : Gain  Gain=Roll.p.thruster1
  Gain1 : Gain  Gain=Roll.p.thruster3
  Gain2 : Gain  Gain=Roll.p.thruster2
  Gain3 : Gain  Gain=Roll_thrust_operator
  Gain4 : Gain  Gain=Roll.p.thruster4
  Multiply : Gain  Gain=gain.Roll.p
  Scope1 : Scope
  Selector1 : Selector  InputPortWidth=3  IndexOptions=Index vector (dialog)  Indices=[1]  OutputSizes=1
  Sum : Sum  Inputs=|+-
  Sum1 : Sum  Inputs=|++++
  To Workspace4 : ToWorkspace  VariableName=momentGeneratedRollPlus  SaveFormat=Timeseries  SampleTime=-1
  arm vec 1 : Constant  Value=Params.arm_vec1
  arm vec 2 : Constant  Value=Params.arm_vec2
  arm vec 3 : Constant  Value=Params.arm_vec3
  arm vec 4 : Constant  Value=Params.arm_vec4
  thrust_1 : Gain  Gain=Params.thrust_vec1
  thrust_2 : Gain  Gain=Params.thrust_vec2
  thrust_3 : Gain  Gain=Params.thrust_vec3
  thrust_4 : Gain  Gain=Params.thrust_vec4
  thruster 1 : Subsystem
  thruster 2 : Subsystem
  thruster 3 : Subsystem
  "thruster 4 " : Subsystem
  Out1 : Outport
  wires:
  "thruster 4 "/1(Thrust_4) -> [Thrust_4]
  Cross Product/1 -> Sum1/3  "torque- thruster 1"
  Cross Product1/1 -> Sum1/4  "torque- thruster 2"
  thruster 3/1(Thrust_1) -> [Thrust_3]
  Gain1/1 -> thruster 3/1(T1)
  Gain2/1 -> thruster 2/1(T1)
  arm vec 1/1 -> Cross Product/1
  Abs2/1 -> thrust_3/1
  [Thrust_2] -> Abs/1
  Sum/1 -> Multiply/1  "delta_w(t)"
  thruster 1/1(Thrust_1) -> [Thrust_1]
  wc/1 -> Selector1/1
  thrust_3/1 -> Cross Product2/2
  [Thrust_3] -> Abs2/1
  thruster 2/1(Thrust_2) -> [Thrust_2]
  w_t_1/1 -> Sum/1
  Gain/1 -> thruster 1/1(T1)
  Multiply/1 -> Gain3/1
  Abs1/1 -> thrust_1/1
  arm vec 3/1 -> Cross Product2/1
  thrust_1/1 -> Cross Product/2
  thrust_2/1 -> Cross Product1/2
  Gain3/1 -> Gain2/1, Gain/1, Gain4/1, Gain1/1  "Thrust required"
  Sum1/1 -> Scope1/1, Out1/1, To Workspace4/1  "Total moment generated in Roll +"
  Abs/1 -> thrust_2/1
  Gain4/1 -> "thruster 4 "/1(T1)
  [Thrust_1] -> Abs1/1
  Selector1/1 -> Sum/2
  thrust_4/1 -> Cross Product3/2
  arm vec 4/1 -> Cross Product3/1
  Cross Product2/1 -> Sum1/2  "torque- thruster  3"
  Abs3/1 -> thrust_4/1
  arm vec 2/1 -> Cross Product1/1
  [Thrust_4] -> Abs3/1
  Cross Product3/1 -> Sum1/1  "torque- thruster  4"

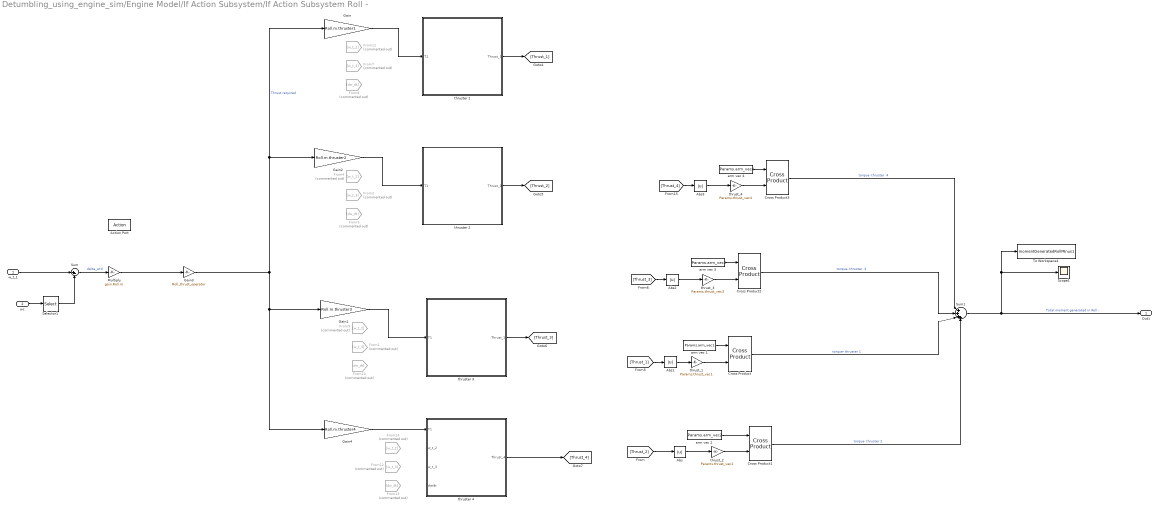
== system Detumbling_using_engine_sim/Engine Model/If Action Subsystem/If Action Subsystem Roll - ==
  w_t_1 : Inport
  wc : Inport  Port=2
  Action Port : ActionPort  ActionPortLabel=else
  Abs{,1..3} (4 alike) : Abs  SaturateOnIntegerOverflow=off
  Cross Product{,1..3} (4 alike) : matrix_library/Cross Product
  From{1..2,7,12} (4 alike) : From  Commented=on  GotoTag=w_t_3
  From{3,8,10,13} (4 alike) : From  Commented=on  GotoTag=dw_dt
  From{4,9,11,14} (4 alike) : From  Commented=on  GotoTag=w_t_2
  Gain : Gain  Gain=Roll.m.thruster1
  Gain1 : Gain  Gain=Roll.m.thruster3
  Gain2 : Gain  Gain=Roll.m.thruster2
  Gain3 : Gain  Gain=Roll_thrust_operator
  Gain4 : Gain  Gain=Roll.m.thruster4
  Multiply : Gain  Gain=gain.Roll.m
  Scope1 : Scope
  Selector1 : Selector  InputPortWidth=3  IndexOptions=Index vector (dialog)  Indices=[1]  OutputSizes=1
  Sum : Sum  Inputs=|+-
  Sum1 : Sum  Inputs=|++++
  To Workspace4 : ToWorkspace  VariableName=momentGeneratedRollMinus1  SaveFormat=Timeseries  SampleTime=-1
  arm vec 1 : Constant  Value=Params.arm_vec1
  arm vec 2 : Constant  Value=Params.arm_vec2
  arm vec 3 : Constant  Value=Params.arm_vec3
  arm vec 4 : Constant  Value=Params.arm_vec4
  thrust_1 : Gain  Gain=Params.thrust_vec1
  thrust_2 : Gain  Gain=Params.thrust_vec2
  thrust_3 : Gain  Gain=Params.thrust_vec3
  thrust_4 : Gain  Gain=Params.thrust_vec4
  thruster 1 : Subsystem
  thruster 2 : Subsystem
  thruster 3 : Subsystem
  "thruster 4 " : Subsystem
  Out1 : Outport
  wires:
  arm vec 1/1 -> Cross Product/1
  Gain2/1 -> thruster 2/1(T1)
  Abs2/1 -> thrust_3/1
  thruster 3/1(Thrust_1) -> [Thrust_3]
  Cross Product1/1 -> Sum1/4  "torque- thruster 2"
  "thruster 4 "/1(Thrust_4) -> [Thrust_4]
  Multiply/1 -> Gain3/1
  arm vec 4/1 -> Cross Product3/1
  Gain1/1 -> thruster 3/1(T1)
  Abs3/1 -> thrust_4/1
  [Thrust_1] -> Abs1/1
  Abs/1 -> thrust_2/1
  Cross Product2/1 -> Sum1/2  "torque- thruster  3"
  arm vec 2/1 -> Cross Product1/1
  Sum1/1 -> To Workspace4/1, Scope1/1, Out1/1  "Total moment generated in Roll -"
  Gain3/1 -> Gain2/1, Gain/1, Gain4/1, Gain1/1  "Thrust required"
  thrust_1/1 -> Cross Product/2
  [Thrust_4] -> Abs3/1
  arm vec 3/1 -> Cross Product2/1
  Gain/1 -> thruster 1/1(T1)
  Cross Product3/1 -> Sum1/1  "torque- thruster  4"
  Cross Product/1 -> Sum1/3  "torque- thruster 1"
  thruster 2/1(Thrust_2) -> [Thrust_2]
  Sum/1 -> Multiply/1  "delta_w(t)"
  [Thrust_3] -> Abs2/1
  wc/1 -> Selector1/1
  w_t_1/1 -> Sum/1
  thruster 1/1(Thrust_1) -> [Thrust_1]
  thrust_3/1 -> Cross Product2/2
  thrust_4/1 -> Cross Product3/2
  [Thrust_2] -> Abs/1
  Abs1/1 -> thrust_1/1
  thrust_2/1 -> Cross Product1/2
  Selector1/1 -> Sum/2
  Gain4/1 -> "thruster 4 "/1(T1)

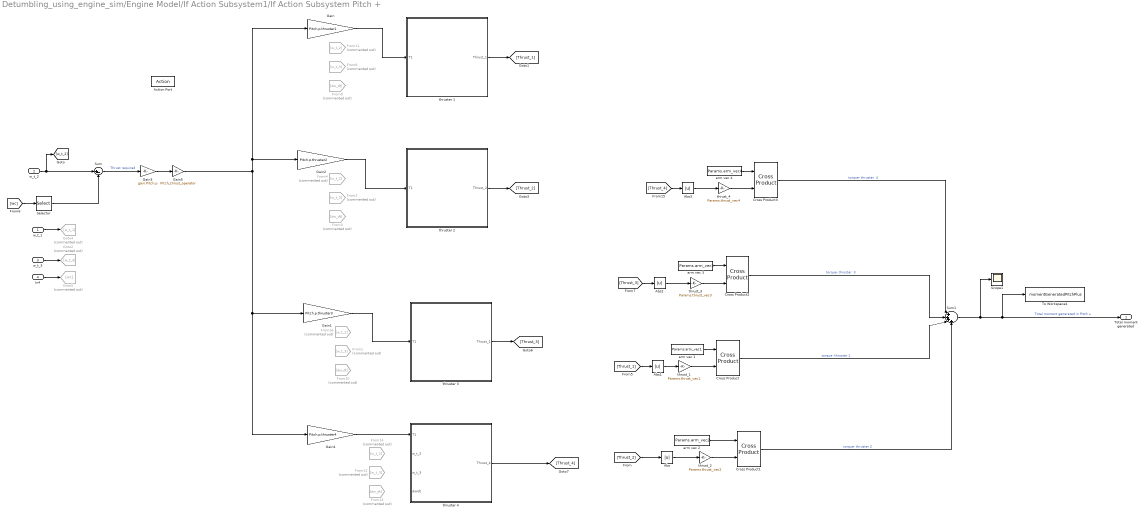
== system Detumbling_using_engine_sim/Engine Model/If Action Subsystem1/If Action Subsystem Pitch + ==
  w_t_1 : Inport
  w_t_2 : Inport  Port=2
  w_t_3 : Inport  Port=3
  In4 : Inport  Port=4
  Action Port : ActionPort  ActionPortLabel=if(u1 > 0)
  Abs{,1..3} (4 alike) : Abs  SaturateOnIntegerOverflow=off
  Cross Product{,1..3} (4 alike) : matrix_library/Cross Product
  From{1..2,8,12} (4 alike) : From  Commented=on  GotoTag=w_t_3
  From{3,9..10,13} (4 alike) : From  Commented=on  GotoTag=dw_dt
  From{4,11,14,16} (4 alike) : From  Commented=on  GotoTag=w_t_2
  Gain : Gain  Gain=Pitch.p.thruster1
  Gain1 : Gain  Gain=Pitch.p.thruster3
  Gain2 : Gain  Gain=Pitch.p.thruster2
  Gain3 : Gain  Gain=gain.Pitch.p
  Gain4 : Gain  Gain=Pitch.p.thruster4
  Gain5 : Gain  Gain=Pitch_thrust_operator
  Goto2 : Goto  Commented=on  GotoTag=w_t_3
  Goto4 : Goto  Commented=on  GotoTag=w_t_1
  Goto5 : Goto  Commented=on  GotoTag=wc
  Scope1 : Scope
  Selector : Selector  InputPortWidth=3  IndexOptions=Index vector (dialog)  Indices=2  OutputSizes=1
  Sum : Sum  Inputs=|+-
  Sum1 : Sum  Inputs=|++++
  To Workspace4 : ToWorkspace  VariableName=momentGeneratedPitchPlus  SaveFormat=Timeseries  SampleTime=-1
  arm vec 1 : Constant  Value=Params.arm_vec1
  arm vec 2 : Constant  Value=Params.arm_vec2
  arm vec 3 : Constant  Value=Params.arm_vec3
  arm vec 4 : Constant  Value=Params.arm_vec4
  thrust_1 : Gain  Gain=Params.thrust_vec1
  thrust_2 : Gain  Gain=Params.thrust_vec2
  thrust_3 : Gain  Gain=Params.thrust_vec3
  thrust_4 : Gain  Gain=Params.thrust_vec4
  thruster 1 : Subsystem
  thruster 2 : Subsystem
  thruster 3 : Subsystem
  "thruster 4 " : Subsystem
  "Total moment generated " : Outport
  wires:
  w_t_1/1 -> Goto4/1
  Selector/1 -> Sum/2
  w_t_2/1 -> Sum/1, [w_t_2]
  w_t_3/1 -> Goto2/1
  In4/1 -> Goto5/1
  [wc] -> Selector/1
  arm vec 1/1 -> Cross Product/1
  Gain2/1 -> thruster 2/1(T1)
  Abs2/1 -> thrust_3/1
  thruster 3/1(Thrust_1) -> [Thrust_3]
  Cross Product1/1 -> Sum1/4  "torque- thruster 2"
  "thruster 4 "/1(Thrust_4) -> [Thrust_4]
  Cross Product3/1 -> Sum1/1  "torque- thruster  4"
  Cross Product/1 -> Sum1/3  "torque- thruster 1"
  arm vec 4/1 -> Cross Product3/1
  Gain1/1 -> thruster 3/1(T1)
  Abs3/1 -> thrust_4/1
  [Thrust_1] -> Abs1/1
  Gain4/1 -> "thruster 4 "/1(T1)
  Abs/1 -> thrust_2/1
  Cross Product2/1 -> Sum1/2  "torque- thruster  3"
  arm vec 2/1 -> Cross Product1/1
  Sum/1 -> Gain3/1  "Thrust required"
  thrust_1/1 -> Cross Product/2
  Sum1/1 -> Scope1/1, "Total moment generated "/1, To Workspace4/1  "Total moment generated in Pitch +"
  [Thrust_4] -> Abs3/1
  Gain/1 -> thruster 1/1(T1)
  arm vec 3/1 -> Cross Product2/1
  thruster 2/1(Thrust_2) -> [Thrust_2]
  [Thrust_3] -> Abs2/1
  thruster 1/1(Thrust_1) -> [Thrust_1]
  thrust_3/1 -> Cross Product2/2
  thrust_4/1 -> Cross Product3/2
  [Thrust_2] -> Abs/1
  Abs1/1 -> thrust_1/1
  thrust_2/1 -> Cross Product1/2
  Gain3/1 -> Gain5/1
  Gain5/1 -> Gain4/1, Gain1/1, Gain2/1, Gain/1

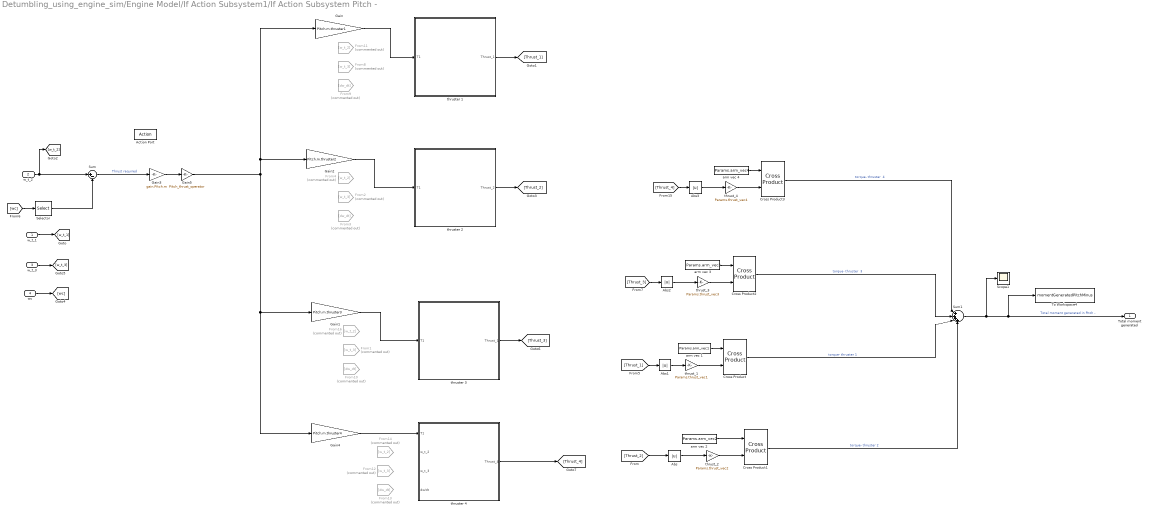
== system Detumbling_using_engine_sim/Engine Model/If Action Subsystem1/If Action Subsystem Pitch - ==
  w_t_1 : Inport
  w_t_2 : Inport  Port=2
  w_t_3 : Inport  Port=3
  wc : Inport  Port=4
  Action Port : ActionPort  ActionPortLabel=else
  Abs{,1..3} (4 alike) : Abs  SaturateOnIntegerOverflow=off
  Cross Product{,1..3} (4 alike) : matrix_library/Cross Product
  From{1..2,8,12} (4 alike) : From  Commented=on  GotoTag=w_t_3
  From{3,9..10,13} (4 alike) : From  Commented=on  GotoTag=dw_dt
  From{4,11,14,16} (4 alike) : From  Commented=on  GotoTag=w_t_2
  Gain : Gain  Gain=Pitch.m.thruster1
  Gain1 : Gain  Gain=Pitch.m.thruster3
  Gain2 : Gain  Gain=Pitch.m.thruster2
  Gain3 : Gain  Gain=gain.Pitch.m
  Gain4 : Gain  Gain=Pitch.m.thruster4
  Gain5 : Gain  Gain=Pitch_thrust_operator
  Scope1 : Scope
  Selector : Selector  InputPortWidth=3  IndexOptions=Index vector (dialog)  Indices=2  OutputSizes=1
  Sum : Sum  Inputs=|+-
  Sum1 : Sum  Inputs=|++++
  To Workspace4 : ToWorkspace  VariableName=momentGeneratedPitchMinus  SaveFormat=Timeseries  SampleTime=-1
  arm vec 1 : Constant  Value=Params.arm_vec1
  arm vec 2 : Constant  Value=Params.arm_vec2
  arm vec 3 : Constant  Value=Params.arm_vec3
  arm vec 4 : Constant  Value=Params.arm_vec4
  thrust_1 : Gain  Gain=Params.thrust_vec1
  thrust_2 : Gain  Gain=Params.thrust_vec2
  thrust_3 : Gain  Gain=Params.thrust_vec3
  thrust_4 : Gain  Gain=Params.thrust_vec4
  thruster 1 : Subsystem
  thruster 2 : Subsystem
  thruster 3 : Subsystem
  "thruster 4 " : Subsystem
  "Total moment generated " : Outport
  wires:
  w_t_1/1 -> [w_t_1]
  w_t_2/1 -> Sum/1, [w_t_2]
  [wc] -> Selector/1
  Selector/1 -> Sum/2
  wc/1 -> [wc]
  w_t_3/1 -> [w_t_3]
  Cross Product/1 -> Sum1/3  "torque- thruster 1"
  thruster 3/1(Thrust_1) -> [Thrust_3]
  arm vec 4/1 -> Cross Product3/1
  Cross Product1/1 -> Sum1/4  "torque- thruster 2"
  arm vec 1/1 -> Cross Product/1
  Gain2/1 -> thruster 2/1(T1)
  [Thrust_2] -> Abs/1
  thrust_2/1 -> Cross Product1/2
  thrust_4/1 -> Cross Product3/2
  thruster 1/1(Thrust_1) -> [Thrust_1]
  [Thrust_3] -> Abs2/1
  thrust_1/1 -> Cross Product/2
  arm vec 3/1 -> Cross Product2/1
  Abs1/1 -> thrust_1/1
  thruster 2/1(Thrust_2) -> [Thrust_2]
  Sum1/1 -> Scope1/1, "Total moment generated "/1, To Workspace4/1  "Total moment generated in Pitch -"
  [Thrust_4] -> Abs3/1
  Gain/1 -> thruster 1/1(T1)
  Cross Product2/1 -> Sum1/2  "torque- thruster  3"
  [Thrust_1] -> Abs1/1
  thrust_3/1 -> Cross Product2/2
  Cross Product3/1 -> Sum1/1  "torque- thruster  4"
  arm vec 2/1 -> Cross Product1/1
  Gain4/1 -> "thruster 4 "/1(T1)
  Abs/1 -> thrust_2/1
  Gain1/1 -> thruster 3/1(T1)
  Abs2/1 -> thrust_3/1
  Gain3/1 -> Gain5/1
  Gain5/1 -> Gain2/1, Gain/1, Gain4/1, Gain1/1
  "thruster 4 "/1(Thrust_4) -> [Thrust_4]
  Sum/1 -> Gain3/1  "Thrust required"
  Abs3/1 -> thrust_4/1

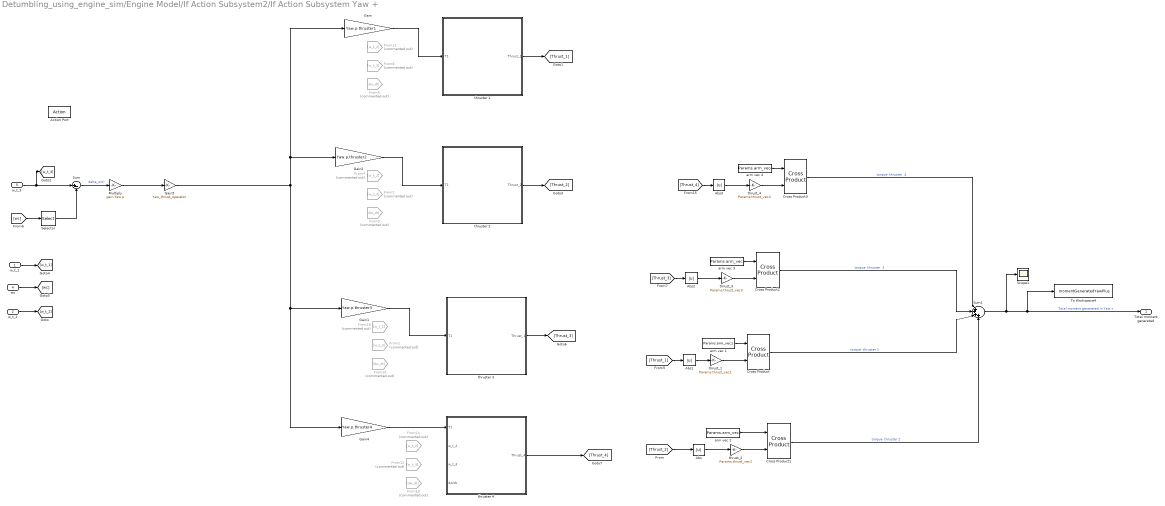
== system Detumbling_using_engine_sim/Engine Model/If Action Subsystem2/If Action Subsystem Yaw + ==
  w_t_1 : Inport
  w_t_2 : Inport  Port=2
  w_t_3 : Inport  Port=3
  wc : Inport  Port=4
  Action Port : ActionPort  ActionPortLabel=if(u1 > 0)
  Abs{,1..3} (4 alike) : Abs  SaturateOnIntegerOverflow=off
  Cross Product{,1..3} (4 alike) : matrix_library/Cross Product
  From{1..2,8,12} (4 alike) : From  Commented=on  GotoTag=w_t_3
  From{3,9..10,13} (4 alike) : From  Commented=on  GotoTag=dw_dt
  From{4,11,14,16} (4 alike) : From  Commented=on  GotoTag=w_t_2
  Gain : Gain  Gain=Yaw.p.thruster1
  Gain1 : Gain  Gain=Yaw.p.thruster3
  Gain2 : Gain  Gain=Yaw.p.thruster2
  Gain4 : Gain  Gain=Yaw.p.thruster4
  Gain5 : Gain  Gain=Yaw_thrust_operator
  Multiply : Gain  Gain=gain.Yaw.p
  Scope1 : Scope
  Selector : Selector  InputPortWidth=3  IndexOptions=Index vector (dialog)  Indices=3  OutputSizes=1
  Sum : Sum  Inputs=|+-
  Sum1 : Sum  Inputs=|++++
  To Workspace4 : ToWorkspace  VariableName=momentGeneratedYawPlus  SaveFormat=Timeseries  SampleTime=-1
  arm vec 1 : Constant  Value=Params.arm_vec1
  arm vec 2 : Constant  Value=Params.arm_vec2
  arm vec 3 : Constant  Value=Params.arm_vec3
  arm vec 4 : Constant  Value=Params.arm_vec4
  thrust_1 : Gain  Gain=Params.thrust_vec1
  thrust_2 : Gain  Gain=Params.thrust_vec2
  thrust_3 : Gain  Gain=Params.thrust_vec3
  thrust_4 : Gain  Gain=Params.thrust_vec4
  thruster 1 : Subsystem
  thruster 2 : Subsystem
  thruster 3 : Subsystem
  "thruster 4 " : Subsystem
  "Total moment generated " : Outport
  wires:
  w_t_1/1 -> [w_t_1]
  Sum/1 -> Multiply/1  "delta_w(t)"
  w_t_2/1 -> [w_t_2]
  w_t_3/1 -> [w_t_3], Sum/1
  Multiply/1 -> Gain5/1
  wc/1 -> [wc]
  [wc] -> Selector/1
  Selector/1 -> Sum/2
  Abs3/1 -> thrust_4/1
  "thruster 4 "/1(Thrust_4) -> [Thrust_4]
  Abs2/1 -> thrust_3/1
  Gain1/1 -> thruster 3/1(T1)
  Abs/1 -> thrust_2/1
  [Thrust_4] -> Abs3/1
  Sum1/1 -> Scope1/1, "Total moment generated "/1, To Workspace4/1  "Total moment generated in Yaw +"
  thrust_1/1 -> Cross Product/2
  arm vec 3/1 -> Cross Product2/1
  Abs1/1 -> thrust_1/1
  [Thrust_3] -> Abs2/1
  thruster 1/1(Thrust_1) -> [Thrust_1]
  Cross Product1/1 -> Sum1/4  "torque- thruster 2"
  Gain2/1 -> thruster 2/1(T1)
  arm vec 1/1 -> Cross Product/1
  thruster 3/1(Thrust_1) -> [Thrust_3]
  thrust_4/1 -> Cross Product3/2
  thrust_2/1 -> Cross Product1/2
  arm vec 4/1 -> Cross Product3/1
  Cross Product/1 -> Sum1/3  "torque- thruster 1"
  Gain4/1 -> "thruster 4 "/1(T1)
  [Thrust_2] -> Abs/1
  Gain5/1 -> Gain4/1, Gain1/1, Gain2/1, Gain/1
  Cross Product3/1 -> Sum1/1  "torque- thruster  4"
  [Thrust_1] -> Abs1/1
  thruster 2/1(Thrust_2) -> [Thrust_2]
  Cross Product2/1 -> Sum1/2  "torque- thruster  3"
  arm vec 2/1 -> Cross Product1/1
  Gain/1 -> thruster 1/1(T1)
  thrust_3/1 -> Cross Product2/2
